simulink model "H4Q"  (R2013b)
settings: Solver=FixedStepDiscrete  SolverMode=SingleTasking  StartTime=0.0  StopTime=0.9  FixedStep=Tpas  RelTol=1e-3
undefined symbols (not defined in the file): fmod4Q, I4Q, KLP4Q, L, P4Q, R, SatPIH4Q, TLP4Q, Tpas, Vdc
libraries: powerlib x9, simulink x7, powerlib_meascontrol x5
settings Model: Creator=LiberT  LastModifiedBy=LiberT
settings DataIOCC: SignalLoggingSaveFormat=ModelDataLogs
settings OptimizationCC: ExpressionDepthLimit=2147483647
settings DebuggingCC: MultiTaskDSMMsg=warning  MultiTaskCondExecSysMsg=none  FcnCallInpInsideContextMsg=EnableAllAsWarning  UnconnectedInputMsg=none  UnconnectedOutputMsg=none  UnconnectedLineMsg=none  StateNameClashWarn=warning
settings RTWCC: IncludeERTFirstTime=on

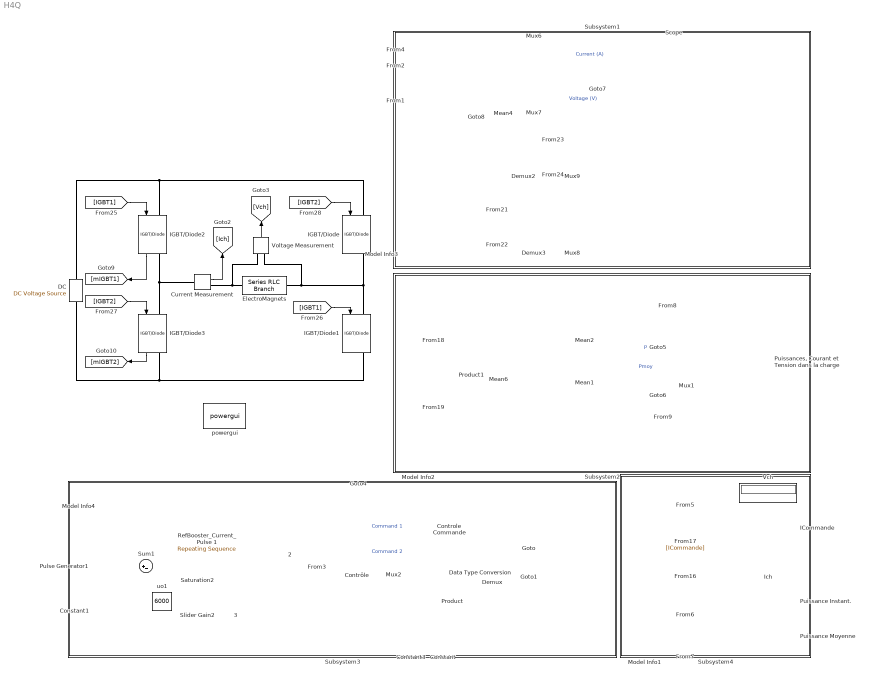
== system H4Q ==
  " 2" : ManualSwitch
  " 3" : ManualSwitch  CurrentSetting=0
  Constant : Constant  Value=[1 1]
  Constant1 : Constant  Value=6000
  Constant3 : Constant  Value=0
  Controle Commande : ManualSwitch
  Contrôle : Subsystem  TreatAsAtomicUnit=on
      settings: MinAlgLoopOccurrences=on
  Current Measurement : powerlib/Measurements/Current Measurement  PhasorSimulation=off  OutputType=Complex  PSBequivalent=0
  DC : powerlib/Electrical Sources/DC Voltage Source  Amplitude=Vdc  Measurements=None
  Data Type Conversion : DataTypeConversion  OutDataTypeStr=boolean
  Demux : Demux  Outputs=2
  Demux2 : Demux  Outputs=2
  Demux3 : Demux  Outputs=2
  "ElectroMagnets " : powerlib/Elements/Series RLC Branch  LConnTagsString=__new0  RConnTagsString=__new0  BranchType=RL  Resistance=R  Inductance=L  SetiL0=off  InitialCurrent=0  Capacitance=1e-6  Setx0=off  InitialVoltage=0  Measurements=Branch voltage and current
  "ICommande " : Display
  IGBT/Diode{,1..3} (4 alike) : powerlib/Power Electronics/IGBT//Diode  Ron=1e-3  Rs=1e5  Cs=inf  Measurements=on
  Ich : Display
  Mean1 : powerlib_meascontrol/Measurements/Mean  Freq=1/.9  Vinit=0  Ts=Tpas
  Mean2 : powerlib_meascontrol/Measurements/Mean  Freq=fmod4Q  Vinit=0  Ts=Tpas
  Mean4 : powerlib_meascontrol/Measurements/Mean  Freq=fmod4Q  Vinit=0  Ts=Tpas
  Mean6 : powerlib_meascontrol/Measurements/Mean  Freq=fmod4Q/2  Vinit=0  Ts=Tpas
  Model Info1 : simulink/Model-Wide Utilities/Model Info  InitialBlockCM=None  BlockCM=None  Frame=on  DisplayStringWithTags=Résultats  HorizontalTextAlignment=Center  LeftAlignmentValue=0.5  SourceBlockDiagram=H4Q  TagMaxNumber=20
  Model Info2 : simulink/Model-Wide Utilities/Model Info  InitialBlockCM=None  BlockCM=None  Frame=on  DisplayStringWithTags=Résultats  HorizontalTextAlignment=Center  LeftAlignmentValue=0.5  SourceBlockDiagram=H4Q  TagMaxNumber=20
  Model Info3 : simulink/Model-Wide Utilities/Model Info  InitialBlockCM=None  BlockCM=None  Frame=on  DisplayStringWithTags=Résultats  HorizontalTextAlignment=Center  LeftAlignmentValue=0.5  SourceBlockDiagram=H4Q  TagMaxNumber=20
  Model Info4 : simulink/Model-Wide Utilities/Model Info  InitialBlockCM=None  BlockCM=None  Frame=on  DisplayStringWithTags=Commande  HorizontalTextAlignment=Center  LeftAlignmentValue=0.5  SourceBlockDiagram=H4Q  TagMaxNumber=20
  Mux{1..2,6..9} (6 alike) : Mux  Inputs=2
  Product : Product
  Product1 : Product
  Puissance Instant. : Display
  Puissance Moyenne : Display
  "Puissances, Courant et Tension dans la charge" : Scope  NumInputPorts=3
      settings: TickLabels=on  TimeRange=0.9  YMin=-100~-25000000~-5000  YMax=6200~25000000~4500
  Pulse Generator1 : DiscretePulseGenerator  Amplitude=12000  Period=floor(.4 /Tpas)  PulseWidth=floor(.4 * .5 / Tpas)  PhaseDelay=floor(.001 / Tpas)  SampleTime=Tpas
  RefBooster_Current_Pulse 1 : simulink/Sources/Repeating Sequence  rep_seq_t="[0 108.51e-3 127.6e-3 132e-3 200e-3 250e-3 283.33e-3 310e-3 366.66e-3  490e-3 533e-3 683.33e-3 900e-3]"  rep_seq_y=[333 333 1000 1031 1500 2000 2500 3000 4000 6000 6000 333 333]
  Saturation2 : Saturate  UpperLimit=5000  LowerLimit=2000
  Scope : Scope  NumInputPorts=6
      settings: TimeRange=0.9  YMin=-7000~-12500~-0.1~-0.1~-7000~-6000  YMax=7000~7500~1.1~1.1~7000~6000  SaveName=hacheur4quadrants  MaxDataPoints=10000
  Slider Gain2 : simulink/Math Operations/Slider Gain  low=0  gain=0.54  high=1
  Subsystem1 : Subsystem
      mask Display: disp('')
  Subsystem2 : Subsystem
      mask Display: disp('')
  Subsystem3 : Subsystem
      mask Display: disp('')
  Subsystem4 : Subsystem
      mask Display: disp('')
  Sum1 : Sum  Inputs=|+-
  Vch : Display
  Voltage Measurement : powerlib/Measurements/Voltage Measurement  PhasorSimulation=off  OutputType=Complex  PSBequivalent=0
  powergui : powerlib/powergui  Priority=1  SimulationMode=Discrete  SolverType=Tustin  SampleTime=Tpas  frequency=60  SPID=on  DisableSnubberDevices=off  DisableRonSwitches=off  DisableVfSwitches=off  SwTol=0  Interpol=off  DisplayEquations=off  frequencyindice=0  Pbase=100e6  ErrMax=1e-4  Iterations=50  UnitsV=kV  UnitsW=MW  FunctionMessages=off  echomessages=off  HookPort=off  EnableUseOfTLC=off  x0status=blocks  RestoreLinks=warning  ResistiveCurrentMeasurement=off  Frange=[0:2:500]  Ylog=off  Xlog=on  ShowGrid=off  save=off  variable=ZData  ZoomFFT=off  StartTime=0.0  cycles=1  DisplayStyle=1  fundamental=60  FreqAxis=off  MaxFrequency=1000  frequencyindicesteady=1  RmsSteady=1  display=off  Ts=0  methode=off
  uo1 : Constant  Value=6000
  wires:
  [Ich] -> Ich/1
  [Vch] -> Vch/1
  [ICommande] -> "ICommande "/1
  [P] -> Puissance Instant./1
  [Pmoy] -> Puissance Moyenne/1
  Constant/1 -> Product/2
  Constant3/1 -> Product/1
  Controle Commande/1 -> Demux/1
  Mux2/1 -> Controle Commande/1
  Demux/1 -> [IGBT1]
  Demux/2 -> [IGBT2]
  Data Type Conversion/1 -> Controle Commande/2
  Product/1 -> Data Type Conversion/1
  " 2"/1 -> [ICommande], Contrôle/1(Iref)
  [Ich] -> Contrôle/2(IL)
  Contrôle/2(C2) -> Mux2/2  "Command 2"
  Contrôle/1(C1) -> Mux2/1  "Command 1"
  uo1/1 -> Slider Gain2/1
  Slider Gain2/1 -> " 3"/2
  Saturation2/1 -> " 3"/1
  Constant1/1 -> Sum1/2
  RefBooster_Current_Pulse 1/1 -> " 2"/1
  " 3"/1 -> " 2"/2
  Pulse Generator1/1 -> Sum1/1
  Sum1/1 -> Saturation2/1
  Mean1/1 -> [Pmoy], Mux1/2  "Pmoy"
  Mean2/1 -> [P], Mux1/1  "P"
  IGBT/Diode2/1 -> [mIGBT1]
  IGBT/Diode3/1 -> [mIGBT2]
  [IGBT1] -> IGBT/Diode2/1
  [IGBT1] -> IGBT/Diode1/1
  [IGBT2] -> IGBT/Diode3/1
  [IGBT2] -> IGBT/Diode/1
  Current Measurement/1 -> [Ich]
  Voltage Measurement/1 -> [Vch]
  Mux6/1 -> [IScope], Scope/1  "Current (A)"
  Mux7/1 -> Scope/2  "Voltage (V)"
  [Ich] -> Mux6/2
  [mIGBT1] -> Demux2/1
  Mean4/1 -> [VMeanLoad], Mux7/2
  [Vch] -> Mux7/1, Mean4/1
  [mIGBT2] -> Demux3/1
  [IGBT1] -> Scope/3
  Mux8/1 -> Scope/6
  Mux9/1 -> Scope/5
  [IGBT2] -> Scope/4
  Demux2/1 -> Mux9/1
  Demux3/1 -> Mux9/2
  Demux2/2 -> Mux8/1
  Demux3/2 -> Mux8/2
  [ICommande] -> Mux6/1
  [Vch] -> Product1/1
  [Ich] -> Product1/2
  Product1/1 -> Mean6/1
  Mean6/1 -> Mean1/1, Mean2/1
  Mux1/1 -> "Puissances, Courant et Tension dans la charge"/2
  [IScope] -> "Puissances, Courant et Tension dans la charge"/1
  [VMeanLoad] -> "Puissances, Courant et Tension dans la charge"/3
  connections:
  IGBT/Diode3/LConn1 -- Current Measurement/LConn1 -- IGBT/Diode2/RConn1
  IGBT/Diode/LConn1 -- DC/RConn1 -- IGBT/Diode2/LConn1
  IGBT/Diode/RConn1 -- IGBT/Diode1/LConn1 -- Voltage Measurement/LConn2 -- "ElectroMagnets "/RConn1
  IGBT/Diode3/RConn1 -- DC/LConn1 -- IGBT/Diode1/RConn1
  Current Measurement/RConn1 -- Voltage Measurement/LConn1 -- "ElectroMagnets "/LConn1

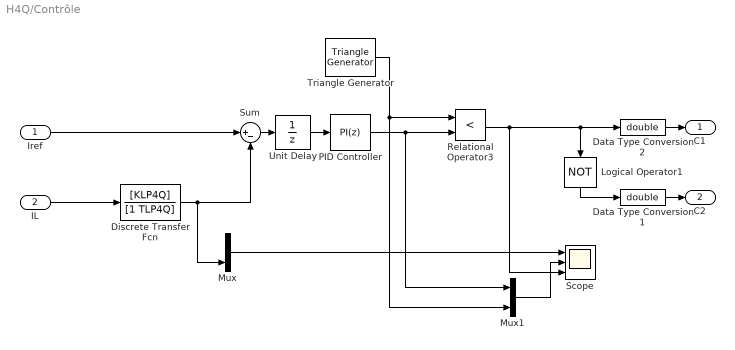
== system H4Q/Contrôle ==
  Iref : Inport
  IL : Inport  Port=2
  Data Type Conversion1 : DataTypeConversion  OutDataTypeStr=double
  Data Type Conversion2 : DataTypeConversion  OutDataTypeStr=double
  Discrete Transfer Fcn : DiscreteTransferFcn  Numerator=[KLP4Q]  Denominator=[1 TLP4Q]
  Logical Operator1 : Logic  Operator=NOT  AllPortsSameDT=off  OutDataTypeStr=boolean
  Mux : Mux  Inputs=2
  Mux1 : Mux  Inputs=2
  PID Controller : simulink/Continuous/PID Controller  Controller=PI  TimeDomain=Discrete-time  SampleTime=Tpas  IntegratorMethod=Forward Euler  FilterMethod=Forward Euler  Form=Parallel  P=P4Q  I=I4Q  D=0  N=100  InitialConditionSource=internal  InitialConditionForIntegrator=0  InitialConditionForFilter=0  ExternalReset=none  LimitOutput=on  UpperSaturationLimit=SatPIH4Q  LowerSaturationLimit=-SatPIH4Q  LinearizeAsGain=on  AntiWindupMode=clamping  Kb=1  TrackingMode=off  Kt=1  PParamMin=[]  PParamMax=[]  IParamMin=[]  IParamMax=[]  DParamMin=[]  DParamMax=[]  NParamMin=[]  NParamMax=[]  KbParamMin=[]  KbParamMax=[]  KtParamMin=[]  KtParamMax=[]  POutMin=[]  POutMax=[]  IOutMin=[]  IOutMax=[]  DOutMin=[]  DOutMax=[]  NOutMin=[]  NOutMax=[]  KbOutMin=[]  KbOutMax=[]  KtOutMin=[]  KtOutMax=[]  IntegratorOutMin=[]  IntegratorOutMax=[]  FilterOutMin=[]  FilterOutMax=[]  SumOutMin=[]  SumOutMax=[]  SumI1OutMin=[]  SumI1OutMax=[]  SumI2OutMin=[]  SumI2OutMax=[]  SumI3OutMin=[]  SumI3OutMax=[]  SumDOutMin=[]  SumDOutMax=[]  SaturationOutMin=[]  SaturationOutMax=[]  IntegratorContinuousStateAttributes=''  IntegratorStateMustResolveToSignalObject=off  IntegratorRTWStateStorageClass=Auto  FilterContinuousStateAttributes=''  FilterStateMustResolveToSignalObject=off  FilterRTWStateStorageClass=Auto
  Relational Operator3 : RelationalOperator  Operator=<  OutDataTypeStr=boolean
  Scope : Scope  NumInputPorts=3
      settings: TimeRange=0.01  YMin=0~-1.2~-5  YMax=6000~1.2~5
  Sum : Sum  Inputs=|+-
  Triangle Generator : powerlib_meascontrol/Pulse & Signal Generators/Triangle Generator  Freq=fmod4Q  Phase=180  Ts=Tpas
  Unit Delay : UnitDelay  SampleTime=-1
  C1 : Outport
  C2 : Outport  Port=2
  wires:
  Triangle Generator/1 -> Mux1/2, Relational Operator3/1
  Relational Operator3/1 -> Logical Operator1/1, Data Type Conversion2/1, Scope/3
  Data Type Conversion2/1 -> C1/1
  Logical Operator1/1 -> Data Type Conversion1/1
  Data Type Conversion1/1 -> C2/1
  Mux/1 -> Scope/1
  Mux1/1 -> Scope/2
  PID Controller/1 -> Relational Operator3/2, Mux1/1
  Discrete Transfer Fcn/1 -> Mux/2, Sum/2
  IL/1 -> Discrete Transfer Fcn/1
  Iref/1 -> Sum/1
  Unit Delay/1 -> PID Controller/1
  Sum/1 -> Unit Delay/1

== system H4Q/Subsystem1 ==

== system H4Q/Subsystem2 ==

== system H4Q/Subsystem3 ==

== system H4Q/Subsystem4 ==
